simulink model "cobaTugas"  (R2018a)
settings: Solver=VariableStepAuto  StartTime=0.0  StopTime=3  RelTol=1e-3
values from neighbouring files (symbols this model uses):
  b = 4e-4    (= 0.0004)    [speed_control_sim.m]    (also in works.m)
  J = 5.4e-5    (= 5.4e-05)    [speed_control_sim.m]    (also in works.m)
  Ka = 6e-5    (= 6e-05)    [speed_control_sim.m]    (also in works.m)
  Kb = 5.4e-2    (= 0.054)    [speed_control_sim.m]    (also in works.m = 0.055)
  Kd = 0.1    [speed_control_sim.m]    (also in works.m = 20)
  Ki = 100    [speed_control_sim.m]    (also in works.m)
  Kp = 20    [speed_control_sim.m]    (also in works.m = 0.1)
  Ks = 1    [works.m]
  L = 0.01-M/40000    (= 0.00935)    [speed_control_sim.m]    (also in works.m = 0.00995)
  R = 0.2+M/2000    (= 0.213)    [speed_control_sim.m]    (also in works.m = 0.201)
  sampTime = 1e-3    (= 0.001)    [works.m]
settings Model: Creator=Thoriqul Aziz  LastModifiedBy=Thoriqul Aziz

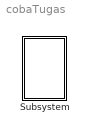
== system cobaTugas ==
  Subsystem : Subsystem

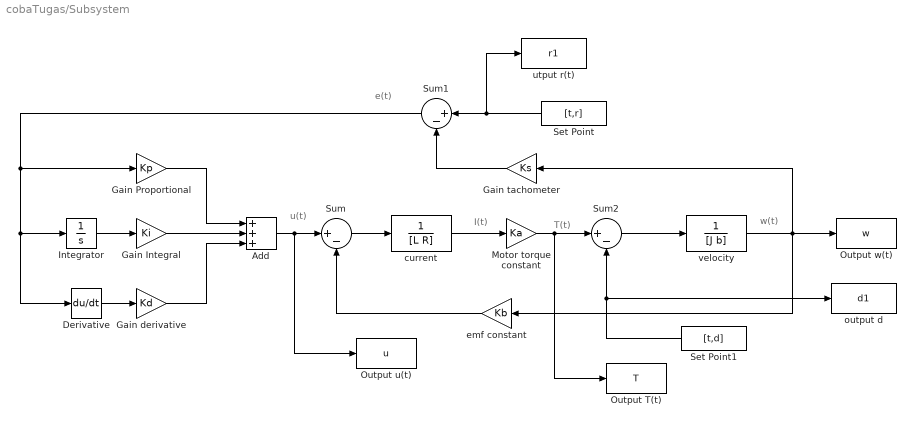
== system cobaTugas/Subsystem ==
  note: I(t)
  note: T(t)
  note: u(t)
  note: w(t)
  note: e(t)
  Add : Sum  Inputs=+++
  Derivative : Derivative
  Gain Integral : Gain  Gain=Ki
  Gain Proportional : Gain  Gain=Kp
  Gain derivative : Gain  Gain=Kd
  Gain tachometer : Gain  Gain=Ks
  Integrator : Integrator
  Motor torque constant : Gain  Gain=Ka
  Output T(t) : ToWorkspace  VariableName=T  SaveFormat=Timeseries  SampleTime=-1
  Output u(t) : ToWorkspace  VariableName=u  SaveFormat=Timeseries  SampleTime=-1
      settings: Save2DSignal=2-D array (concatenate along first dimension)
  Output w(t) : ToWorkspace  VariableName=w  SaveFormat=Timeseries  SampleTime=-1
  Set Point : FromWorkspace  VariableName=[t,r]  OutDataTypeStr=double  SampleTime=sampTime  OutputAfterFinalValue=Holding final value
  Set Point1 : FromWorkspace  VariableName=[t,d]  OutDataTypeStr=double  SampleTime=sampTime  OutputAfterFinalValue=Holding final value
  Sum : Sum  Inputs=|+-
  Sum1 : Sum  Inputs=|+-
  Sum2 : Sum  Inputs=|+-
  current : TransferFcn  Denominator=[L R]  ContinuousStateAttributes='kirchof'
  emf constant : Gain  Gain=Kb
  output d : ToWorkspace  VariableName=d1  SaveFormat=Timeseries  SampleTime=-1
      settings: Save2DSignal=2-D array (concatenate along first dimension)
  utput r(t) : ToWorkspace  VariableName=r1  SaveFormat=Timeseries  SampleTime=-1
      settings: Save2DSignal=2-D array (concatenate along first dimension)
  "velocity " : TransferFcn  Denominator=[J b]  ContinuousStateAttributes='Newton'
  wires:
  current/1 -> Motor torque constant/1
  "velocity "/1 -> emf constant/1, Gain tachometer/1, Output w(t)/1
  Sum/1 -> current/1
  emf constant/1 -> Sum/2
  Gain tachometer/1 -> Sum1/2
  Set Point/1 -> utput r(t)/1, Sum1/1
  Sum1/1 -> Gain Proportional/1, Derivative/1, Integrator/1
  Integrator/1 -> Gain Integral/1
  Derivative/1 -> Gain derivative/1
  Gain Proportional/1 -> Add/1
  Gain Integral/1 -> Add/2
  Gain derivative/1 -> Add/3
  Add/1 -> Output u(t)/1, Sum/1
  Motor torque constant/1 -> Output T(t)/1, Sum2/1
  Sum2/1 -> "velocity "/1
  Set Point1/1 -> output d/1, Sum2/2
